simulink library "SMXL"  (Simulink 2.3)
libraries: smxl x55, SMXL x9, simulink3 x4
(part 1 of 2)
settings Model: LastModifiedBy=campa

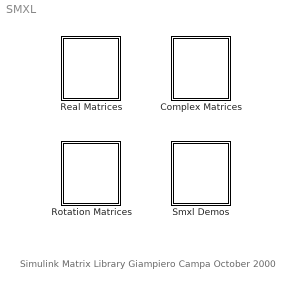
== system SMXL ==
  note: Simulink Matrix Library
      | Giampiero Campa
      | October 2000
  Complex Matrices : Subsystem
      mask Display: disp('Complex\nMatrices')
  Real Matrices : Subsystem
      mask Display: disp('Real\nMatrices')
  Rotation Matrices : Subsystem
      mask Display: disp('R3\nRotation\nMatrices')
  Smxl Demos : Subsystem
      settings: OpenFcn=smxlexamplespath=which('smxl');path(path,[ smxlexamplespath(1:length(smxlexamplespath)-8) 'examples' ]);clear smxlexamplespath;smxldemo
      mask Display: disp('Smxl\nDemos')

== system SMXL/Complex Matrices ==
  note: COMPLEX (AND REAL) MATRICES
  note: Multiplication, Transposition, Pseudoinversion, Rank, Pseudo Singular Values Decomposition
  note: Horizontal Composition, Horizontal Split, Vertical Composition, Vertical Split
  vchcomp : Subsystem  mask(Simulink Matrix Library Block){dims=[3 2 2]}
      mask prompts: dims "[p n m]"
      mask help:
      | Complex Varying Matrices Horizontal Composition
      |   Input 1   : elements of matrix X (p by n)
      |   Input 2   : elements of matrix Y (p by m)
      |   Output   : elements of matrix [X Y] (p by m+n)
      mask Help:
      | <p>
      | Elements of input and output matrices are taken columnwise.
      | </p>
      | <p>
      | To use this block you should have the smxl library in your path.
      | </p>
      mask Display: disp('Z=[X,Y]')
  vchsplit : Subsystem  mask(Simulink Matrix Library Block){dims=[3 2 2]}
      mask prompts: dims "[p n m]"
      mask help:
      | Complex Varying Matrix Horizontal Split
      |   Input       : elements of matrix [X Y] (p by n+m)
      |   Output 1 : elements of matrix X (p by n)
      |   Output 2 : elements of matrix Y (p by m)
      mask Help:
      | <p>
      | Elements of input and output matrices are taken columnwise.
      | </p>
      | <p>
      | To use this block you should have the smxl library in your path.
      | </p>
      mask Display: disp('[X,Y]=Z')
  vcmult : Subsystem  mask(Simulink Matrix Library Block){d=[2 3 2]}
      mask prompts: d "[n p m]"
      mask help:
      | Complex Varying Matrices Multiplication
      |   Input 1   : elements of matrix X (n by p)
      |   Input 2   : elements of matrix Y (p by m)
      |   Output   : elements of matrix X*Y (n by m)
      mask Help:
      | <p>
      | Elements of input and output matrices are taken columnwise.
      | </p>
      | <p>
      | To use this block you should have the smxl library in your path.
      | </p>
      mask Display: disp('Z=X*Y')
  vcpinv : Subsystem  mask(Simulink Matrix Library Block){d=[3 2], tol=1}
      mask prompts: d "[n m]"
      mask help:
      | Complex Varying Matrix Pseudoinversion
      |   Input      : elements of matrix X (n by m)
      |   Output   : elements of matrix Pinv(X) (m by n)
      |   Tol         : tolerance is set to max(m,n)*max(svd(X))*eps*tol
      mask Help:
      | <p>
      | Elements of input and output matrices are taken columnwise.
      | </p>
      | <p>
      | To use this block you should have the smxl library in your path.
      | </p>
      mask Display: disp('Y=pinv(X)')
  vcpsvd : Subsystem  mask(Simulink Matrix Library Block){d=[2 3]}
      mask prompts: d "[n m]"
      mask help:
      | Complex Varying Matrix SVD
      |   Input       : elements of matrix X=USV', (n by m)
      |   Output 1 : elements of matrix U, (n by min(n,m))
      |   Output 2 : elements of matrix S, (square min(n,m))
      |   Output 3 : elements of matrix V, (m by min(n,m))
      |
      |   NOTE     : This is actually a pseudo-svd, since each singular value is
      |                     repeated twice along S diagonal. To have a pure svd just
      |                     pick up every singular value once with the respective
      |                     left and right singular vectors multiplied by sqrt(2).
      mask Help:
      | <p>
      | Elements of input and output matrices are taken columnwise.
      | </p>
      | <p>
      | NOTE     : This is actually a pseudo-svd, since each singular value is
      |                   repeated twice along S diagonal. To have a pure svd just
      |                   pick up every singular value once with the respective
      |                   left and right singular vectors multiplied by sqrt(2).
      | 
      | </p>
      | <p>
      | To use this block you should have the smxl library in your path.
      | </p>
      mask Display: disp('[U,S,V]=svd(X)')
  vcrank : Subsystem  mask(Simulink Matrix Library Block){d=[4 3], tol=1}
      mask prompts: d "[n m]"
      mask help:
      | Complex Varying Matrix Rank
      |   Input      : elements of matrix X (n by m)
      |   Output   : rank of matrix X
      |   Tol         : tolerance is set to max(m,n)*max(svd(X))*eps*tol
      mask Help:
      | <p>
      | Elements of input and output matrices are taken columnwise.
      | </p>
      | <p>
      | To use this block you should have the smxl library in your path.
      | </p>
      mask Display: disp('rank(X)')
  vctrsp : Subsystem  mask(Simulink Matrix Library Block){d=[3 2], h=on}
      mask prompts: d "[n m]"; h "Hermitian"
      mask help:
      | Complex Varying Matrix Transposition
      |   Input      : elements of matrix X (n by m)
      |   Output   : elements of matrix X' (m by n)
      mask Help:
      | <p>
      | Elements of input and output matrices are taken columnwise.
      | </p>
      | <p>
      | To use this block you should have the smxl library in your path.
      | </p>
      mask Display: disp('Y=X''')
  vcvcomp : Subsystem  mask(Simulink Matrix Library Block){dims=[3 3 2]}
      mask prompts: dims "[n m p]"
      mask help:
      | Complex Varying Matrices Vertical Composition
      |   Input 1 : elements of matrix X (n by p)
      |   Input 2 : elements of matrix Y (m by p)
      |   Output : elements of matrix [X;Y] (m+n by p)
      mask Help:
      | <p>
      | Elements of input and output matrices are taken columnwise.
      | </p>
      | <p>
      | To use this block you should have the smxl library in your path.
      | </p>
      mask Display: disp('Z=[X;Y]')
  vcvsplit : Subsystem  mask(Simulink Matrix Library Block){dims=[3 3 2]}
      mask prompts: dims "[n m p]"
      mask help:
      | Complex Varying Matrix Vertical Split
      |   Input       : elements of matrix [X;Y] (n+m by p)
      |   Output 1 : elements of matrix X (n by p)
      |   Output 2 : elements of matrix Y (m by p)
      mask Help:
      | <p>
      | Elements of input and output matrices are taken columnwise.
      | </p>
      | <p>
      | To use this block you should have the smxl library in your path.
      | </p>
      mask Display: disp('[X;Y]=Z')

== system SMXL/Real Matrices ==
  note: Multiplication, Transposition, Pseudoinversion, Rank, Singular Values Decomposition
  note: REAL MATRICES ONLY
  note: Horizontal Composition, Horizontal Split, Vertical Composition, Vertical Split
  vrhcomp : Subsystem  mask(Simulink Matrix Library Block){dims=[3 2 2]}
      mask prompts: dims "[p n m]"
      mask help:
      | Real Varying Matrices Horizontal Composition
      |   Input 1   : elements of matrix X (p by n)
      |   Input 2   : elements of matrix Y (p by m)
      |   Output   : elements of matrix [X Y] (p by m+n)
      mask Help:
      | <p>
      | Elements of input and output matrices are taken columnwise.
      | </p>
      | <p>
      | To use this block you should have the smxl library in your path.
      | </p>
      mask Display: disp('Z=[X,Y]')
  vrhsplit : Subsystem  mask(Simulink Matrix Library Block){dims=[3 2 2]}
      mask prompts: dims "[p n m]"
      mask help:
      | Real Varying Matrix Horizontal Split
      |   Input       : elements of matrix [X Y] (p by n+m)
      |   Output 1 : elements of matrix X (p by n)
      |   Output 2 : elements of matrix Y (p by m)
      mask Help:
      | <p>
      | Elements of input and output matrices are taken columnwise.
      | </p>
      | <p>
      | To use this block you should have the smxl library in your path.
      | </p>
      mask Display: disp('[X,Y]=Z')
  vrmult : S-Function  FunctionName=vrmult  Parameters=dims  PortCounts=[]  SFunctionModules=''  mask(Simulink Matrix Library Block){dims=[2 4 3]}
      mask prompts: dims "[n p m]"
      mask help:
      | Real Varying Matrices Multiplication
      |   Input 1   : elements of matrix X (n by p)
      |   Input 2   : elements of matrix Y (p by m)
      |   Output   : elements of matrix X*Y (n by m)
      mask Help:
      | <p>
      | Elements of input and output matrices are taken columnwise.
      | </p>
      | <p>
      | To use this block you should have the smxl library in your path.
      | </p>
      mask Display: disp('Z=X*Y')
  vrpinv : S-Function  FunctionName=vrpinv  Parameters=dims,tol  PortCounts=[]  SFunctionModules=''  mask(Simulink Matrix Library Block){dims=[3 2], tol=1}
      mask prompts: dims "[n m]"
      mask help:
      | Real Varying Matrix Pseudoinversion
      |   Input      : elements of matrix X (n by m)
      |   Output   : elements of matrix Pinv(X) (m by n)
      |   Tol         : tolerance is set to max(m,n)*max(svd(X))*eps*tol
      mask Help:
      | <p>
      | Elements of input and output matrices are taken columnwise.
      | </p>
      | <p>
      | To use this block you should have the smxl library in your path.
      | </p>
      mask Display: disp('Y=pinv(X)')
  vrrank : Subsystem  mask(Simulink Matrix Library Block){dims=[4 3], tol=1}
      mask prompts: dims "[n m]"
      mask help:
      | Real Varying Matrix Rank
      |   Input      : elements of matrix X (n by m)
      |   Output   : rank of matrix X
      |   Tol         : tolerance is set to max(m,n)*max(svd(X))*eps*tol
      mask Help:
      | <p>
      | Elements of input and output matrices are taken columnwise.
      | </p>
      | <p>
      | To use this block you should have the smxl library in your path.
      | </p>
      mask Display: disp('rank(X)')
  vrsvd : S-Function  FunctionName=vrsvd  Parameters=dims  PortCounts=[]  SFunctionModules=''  mask(Simulink Matrix Library Block){dims=[2 3]}
      mask prompts: dims "[n m]"
      mask help:
      | Real Varying Matrix SVD
      |   Input       : elements of matrix X=USV', (n by m)
      |   Output 1 : elements of matrix U, (n by min(n,m))
      |   Output 2 : elements of matrix S, (square min(n,m))
      |   Output 3 : elements of matrix V, (m by min(n,m))
      mask Help:
      | <p>
      | Elements of input and output matrices are taken columnwise.
      | </p>
      | <p>
      | To use this block you should have the smxl library in your path.
      | </p>
      mask Display: disp('[U,S,V]=svd(X)')
  vrtrsp : Subsystem  mask(Simulink Matrix Library Block){dims=[3 2]}
      mask prompts: dims "[n m]"
      mask help:
      | Real Varying Matrix Transposition
      |   Input      : elements of matrix X (n by m)
      |   Output   : elements of matrix X' (m by n)
      mask Help:
      | <p>
      | Elements of input and output matrices are taken columnwise.
      | </p>
      | <p>
      | To use this block you should have the smxl library in your path.
      | </p>
      mask Display: disp('Y=X''')
  vrvcomp : Subsystem  mask(Simulink Matrix Library Block){dims=[3 3 2]}
      mask prompts: dims "[n m p]"
      mask help:
      | Real Varying Matrices Vertical Composition
      |   Input 1 : elements of matrix X (n by p)
      |   Input 2 : elements of matrix Y (m by p)
      |   Output : elements of matrix [X;Y] (m+n by p)
      mask Help:
      | <p>
      | Elements of input and output matrices are taken columnwise.
      | </p>
      | <p>
      | To use this block you should have the smxl library in your path.
      | </p>
      mask Display: disp('Z=[X;Y]')
  vrvsplit : Subsystem  mask(Simulink Matrix Library Block){dims=[3 3 2]}
      mask prompts: dims "[n m p]"
      mask help:
      | Real Varying Matrix Vertical Split
      |   Input       : elements of matrix [X;Y] (n+m by p)
      |   Output 1 : elements of matrix X (n by p)
      |   Output 2 : elements of matrix Y (m by p)
      mask Help:
      | <p>
      | Elements of input and output matrices are taken columnwise.
      | </p>
      | <p>
      | To use this block you should have the smxl library in your path.
      | </p>
      mask Display: disp('[X;Y]=Z')

== system SMXL/Rotation Matrices ==
  note: Rotation Matrices Library
      | G. Campa & F. Giulietti
      | February 1999
  Euler : Subsystem
      mask Display: disp('Euler')
  Quaternions : Subsystem
      mask Display: disp('Quat')

== system SMXL/Smxl Demos ==

== system SMXL/Complex Matrices/vchcomp ==
  In1 : Inport  Port=1  PortWidth=-1  SampleTime=-1  DataType=auto
      settings: SignalType=auto
  In2 : Inport  Port=2  PortWidth=-1  SampleTime=-1  DataType=auto
      settings: SignalType=auto
  Mux : Mux  Inputs=[dims(1)*dims(2) dims(1)*dims(3)]
  Out1 : Outport  Port=1
  wires:
  In1/1 -> Mux/1
  Mux/1 -> Out1/1
  In2/1 -> Mux/2

== system SMXL/Complex Matrices/vchsplit ==
  In1 : Inport  Port=1  PortWidth=-1  SampleTime=-1  DataType=auto
      settings: SignalType=auto
  Demux : Demux  Outputs=[dims(1)*dims(2) dims(1)*dims(3)]
  Out1 : Outport  Port=1
  Out2 : Outport  Port=2
  wires:
  In1/1 -> Demux/1
  Demux/2 -> Out2/1
  Demux/1 -> Out1/1

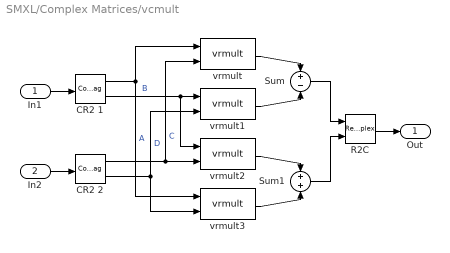
== system SMXL/Complex Matrices/vcmult ==
  In1 : Inport  Port=1  PortWidth=-1  SampleTime=-1  DataType=auto
      settings: SignalType=auto
  In2 : Inport  Port=2  PortWidth=-1  SampleTime=-1  DataType=auto
      settings: SignalType=auto
  CR2 1 : ComplexToRealImag  Output=RealAndImag
  CR2 2 : ComplexToRealImag  Output=RealAndImag
  R2C : RealImagToComplex  Input=RealAndImag  ConstantPart=0
  Sum : Sum  Inputs=+|-  SaturateOnIntegerOverflow=on
  Sum1 : Sum  Inputs=+|+  SaturateOnIntegerOverflow=on
  vrmult{,1..3} (4 alike) : smxl/Real Matrices/vrmult  dims=d
  Out : Outport  Port=1
  wires:
  CR2 1/1 -> vrmult/1, vrmult3/1  "A"
  CR2 1/2 -> vrmult1/1, vrmult2/1  "B"
  CR2 2/2 -> vrmult3/2, vrmult1/2  "D"
  CR2 2/1 -> vrmult2/2, vrmult/2  "C"
  Sum/1 -> R2C/1
  Sum1/1 -> R2C/2
  In1/1 -> CR2 1/1
  R2C/1 -> Out/1
  In2/1 -> CR2 2/1
  vrmult3/1 -> Sum1/2
  vrmult2/1 -> Sum1/1
  vrmult1/1 -> Sum/2
  vrmult/1 -> Sum/1

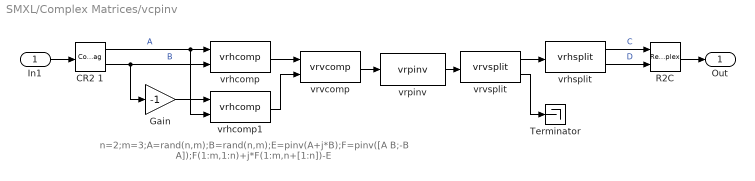
== system SMXL/Complex Matrices/vcpinv ==
  note: n=2;m=3;A=rand(n,m);B=rand(n,m);E=pinv(A+j*B);F=pinv([A B;-B A]);F(1:m,1:n)+j*F(1:m,n+[1:n])-E
  In1 : Inport  Port=1  PortWidth=-1  SampleTime=-1  DataType=auto
      settings: SignalType=auto
  CR2 1 : ComplexToRealImag  Output=RealAndImag
  Gain : Gain  Gain=-1  SaturateOnIntegerOverflow=on
  R2C : RealImagToComplex  Input=RealAndImag  ConstantPart=0
  Terminator : Terminator
  vrhcomp : smxl/Real Matrices/vrhcomp  dims=[d(1) d(2) d(2)]
  vrhcomp1 : smxl/Real Matrices/vrhcomp  dims=[d(1) d(2) d(2)]
  vrhsplit : smxl/Real Matrices/vrhsplit  dims=[d(2) d(1) d(1)]
  vrpinv : smxl/Real Matrices/vrpinv  dims=2*d  tol=tol
  vrvcomp : smxl/Real Matrices/vrvcomp  dims=[d(1) d(1) 2*d(2)]
  vrvsplit : smxl/Real Matrices/vrvsplit  dims=[d(2) d(2) 2*d(1)]
  Out : Outport  Port=1
  wires:
  In1/1 -> CR2 1/1
  CR2 1/1 -> vrhcomp/1, vrhcomp1/2  "A"
  CR2 1/2 -> vrhcomp/2, Gain/1  "B"
  vrhcomp/1 -> vrvcomp/1
  vrhcomp1/1 -> vrvcomp/2
  vrvcomp/1 -> vrpinv/1
  vrpinv/1 -> vrvsplit/1
  vrvsplit/1 -> vrhsplit/1
  vrhsplit/1 -> R2C/1  "C"
  vrhsplit/2 -> R2C/2  "D"
  vrvsplit/2 -> Terminator/1
  Gain/1 -> vrhcomp1/1
  R2C/1 -> Out/1

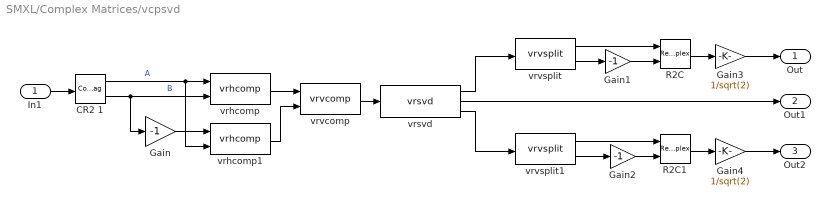
== system SMXL/Complex Matrices/vcpsvd ==
  In1 : Inport  Port=1  PortWidth=-1  SampleTime=-1  DataType=auto
      settings: SignalType=auto
  CR2 1 : ComplexToRealImag  Output=RealAndImag
  Gain : Gain  Gain=-1  SaturateOnIntegerOverflow=on
  Gain1 : Gain  Gain=-1  SaturateOnIntegerOverflow=on
  Gain2 : Gain  Gain=-1  SaturateOnIntegerOverflow=on
  Gain3 : Gain  Gain=1/sqrt(2)  SaturateOnIntegerOverflow=on
  Gain4 : Gain  Gain=1/sqrt(2)  SaturateOnIntegerOverflow=on
  R2C : RealImagToComplex  Input=RealAndImag  ConstantPart=0
  R2C1 : RealImagToComplex  Input=RealAndImag  ConstantPart=0
  vrhcomp : smxl/Real Matrices/vrhcomp  dims=[d(1) d(2) d(2)]
  vrhcomp1 : smxl/Real Matrices/vrhcomp  dims=[d(1) d(2) d(2)]
  vrsvd : smxl/Real Matrices/vrsvd  dims=2*d
  vrvcomp : smxl/Real Matrices/vrvcomp  dims=[d(1) d(1) 2*d(2)]
  vrvsplit : smxl/Real Matrices/vrvsplit  dims=[d(1) d(1) 2*min(d(1),d(2))]
  vrvsplit1 : smxl/Real Matrices/vrvsplit  dims=[d(2) d(2) 2*min(d(1),d(2))]
  Out : Outport  Port=1
  Out1 : Outport  Port=2
  Out2 : Outport  Port=3
  wires:
  In1/1 -> CR2 1/1
  CR2 1/1 -> vrhcomp/1, vrhcomp1/2  "A"
  CR2 1/2 -> vrhcomp/2, Gain/1  "B"
  vrvcomp/1 -> vrsvd/1
  Gain/1 -> vrhcomp1/1
  vrsvd/2 -> Out1/1
  vrsvd/1 -> vrvsplit/1
  vrvsplit/2 -> Gain1/1
  Gain1/1 -> R2C/2
  vrvsplit/1 -> R2C/1
  vrsvd/3 -> vrvsplit1/1
  vrvsplit1/2 -> Gain2/1
  Gain2/1 -> R2C1/2
  vrvsplit1/1 -> R2C1/1
  R2C/1 -> Gain3/1
  Gain3/1 -> Out/1
  R2C1/1 -> Gain4/1
  Gain4/1 -> Out2/1
  vrhcomp/1 -> vrvcomp/1
  vrhcomp1/1 -> vrvcomp/2

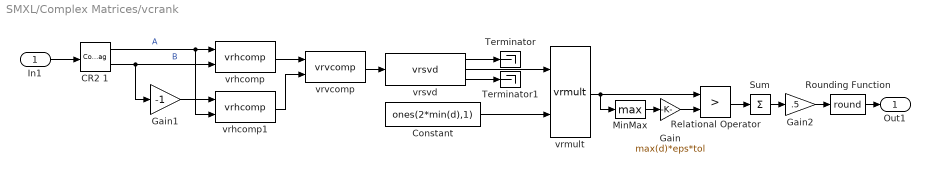
== system SMXL/Complex Matrices/vcrank ==
  In1 : Inport  Port=1  PortWidth=-1  SampleTime=-1  DataType=auto
      settings: SignalType=auto
  CR2 1 : ComplexToRealImag  Output=RealAndImag
  Constant : Constant  Value=ones(2*min(d),1)
  Gain : Gain  Gain=max(d)*eps*tol  SaturateOnIntegerOverflow=on
  Gain1 : Gain  Gain=-1  SaturateOnIntegerOverflow=on
  Gain2 : Gain  Gain=.5  SaturateOnIntegerOverflow=on
  MinMax : MinMax  Function=max  Inputs=1
  Relational Operator : RelationalOperator  Operator=>
  Rounding Function : Rounding  Operator=round
  Sum : Sum  Inputs=1  SaturateOnIntegerOverflow=on
  Terminator : Terminator
  Terminator1 : Terminator
  vrhcomp : smxl/Real Matrices/vrhcomp  dims=[d(1) d(2) d(2)]
  vrhcomp1 : smxl/Real Matrices/vrhcomp  dims=[d(1) d(2) d(2)]
  vrmult : smxl/Real Matrices/vrmult  dims=[2*min(d) 2*min(d) 1]
  vrsvd : smxl/Real Matrices/vrsvd  dims=2*d
  vrvcomp : smxl/Real Matrices/vrvcomp  dims=[d(1) d(1) 2*d(2)]
  Out1 : Outport  Port=1
  wires:
  CR2 1/2 -> vrhcomp/2, Gain1/1  "B"
  CR2 1/1 -> vrhcomp/1, vrhcomp1/2  "A"
  In1/1 -> CR2 1/1
  Gain1/1 -> vrhcomp1/1
  vrvcomp/1 -> vrsvd/1
  Gain/1 -> Relational Operator/2
  MinMax/1 -> Gain/1
  vrmult/1 -> MinMax/1, Relational Operator/1
  vrsvd/2 -> vrmult/1
  Constant/1 -> vrmult/2
  vrsvd/3 -> Terminator1/1
  vrsvd/1 -> Terminator/1
  Relational Operator/1 -> Sum/1
  Rounding Function/1 -> Out1/1
  Gain2/1 -> Rounding Function/1
  Sum/1 -> Gain2/1
  vrhcomp1/1 -> vrvcomp/2
  vrhcomp/1 -> vrvcomp/1

== system SMXL/Complex Matrices/vctrsp ==
  In1 : Inport  Port=1  PortWidth=-1  SampleTime=-1  DataType=auto
      settings: SignalType=auto
  CR2 1 : ComplexToRealImag  Output=RealAndImag
  Gain : Gain  Gain=1-2*h  SaturateOnIntegerOverflow=on
  R2C : RealImagToComplex  Input=RealAndImag  ConstantPart=0
  vrtrsp : smxl/Real Matrices/vrtrsp  dims=d
  vrtrsp1 : smxl/Real Matrices/vrtrsp  dims=d
  Out : Outport  Port=1
  wires:
  In1/1 -> CR2 1/1
  CR2 1/2 -> vrtrsp1/1  "B"
  CR2 1/1 -> vrtrsp/1  "A"
  R2C/1 -> Out/1
  vrtrsp/1 -> R2C/1
  vrtrsp1/1 -> Gain/1
  Gain/1 -> R2C/2

== system SMXL/Complex Matrices/vcvcomp ==
  In1 : Inport  Port=1  PortWidth=-1  SampleTime=-1  DataType=auto
      settings: SignalType=auto
  In2 : Inport  Port=2  PortWidth=-1  SampleTime=-1  DataType=auto
      settings: SignalType=auto
  Mux : Mux  Inputs=[dims(3)*dims(1) dims(3)*dims(2)]
  vctrsp : smxl/Complex Matrices/vctrsp  d=[dims(1) dims(3)]  h=on
  vctrsp1 : smxl/Complex Matrices/vctrsp  d=[dims(2) dims(3)]  h=on
  vctrsp2 : smxl/Complex Matrices/vctrsp  d=[dims(3) dims(2)+dims(1)]  h=on
  Out1 : Outport  Port=1
  wires:
  In1/1 -> vctrsp/1
  In2/1 -> vctrsp1/1
  vctrsp2/1 -> Out1/1
  Mux/1 -> vctrsp2/1
  vctrsp1/1 -> Mux/2
  vctrsp/1 -> Mux/1

== system SMXL/Complex Matrices/vcvsplit ==
  In1 : Inport  Port=1  PortWidth=-1  SampleTime=-1  DataType=auto
      settings: SignalType=auto
  Demux : Demux  Outputs=[dims(3)*dims(1) dims(3)*dims(2)]
  vctrsp : smxl/Complex Matrices/vctrsp  d=[dims(3) dims(1)]  h=on
  vctrsp1 : smxl/Complex Matrices/vctrsp  d=[dims(3) dims(2)]  h=on
  vctrsp2 : smxl/Complex Matrices/vctrsp  d=[dims(2)+dims(1) dims(3)]  h=on
  Out1 : Outport  Port=1
  Out2 : Outport  Port=2
  wires:
  In1/1 -> vctrsp2/1
  vctrsp2/1 -> Demux/1
  Demux/1 -> vctrsp/1
  vctrsp/1 -> Out1/1
  Demux/2 -> vctrsp1/1
  vctrsp1/1 -> Out2/1

== system SMXL/Real Matrices/vrhcomp ==
  In1 : Inport  Port=1  PortWidth=-1  SampleTime=-1  DataType=auto
      settings: SignalType=auto
  In2 : Inport  Port=2  PortWidth=-1  SampleTime=-1  DataType=auto
      settings: SignalType=auto
  Mux : Mux  Inputs=[dims(1)*dims(2) dims(1)*dims(3)]
  Out1 : Outport  Port=1
  wires:
  In2/1 -> Mux/2
  Mux/1 -> Out1/1
  In1/1 -> Mux/1

== system SMXL/Real Matrices/vrhsplit ==
  In1 : Inport  Port=1  PortWidth=-1  SampleTime=-1  DataType=auto
      settings: SignalType=auto
  Demux : Demux  Outputs=[dims(1)*dims(2) dims(1)*dims(3)]
  Out1 : Outport  Port=1
  Out2 : Outport  Port=2
  wires:
  Demux/1 -> Out1/1
  Demux/2 -> Out2/1
  In1/1 -> Demux/1

== system SMXL/Real Matrices/vrrank ==
  In1 : Inport  Port=1  PortWidth=-1  SampleTime=-1  DataType=auto
      settings: SignalType=auto
  Constant : Constant  Value=ones(min(dims),1)
  Gain : Gain  Gain=max(dims)*eps*tol  SaturateOnIntegerOverflow=on
  MinMax : MinMax  Function=max  Inputs=1
  Relational Operator : RelationalOperator  Operator=>
  Sum : Sum  Inputs=1  SaturateOnIntegerOverflow=on
  Terminator : Terminator
  Terminator1 : Terminator
  vrmult : SMXL/Real Matrices/vrmult  dims=[min(dims) min(dims) 1]
  vrsvd : SMXL/Real Matrices/vrsvd  dims=dims
  Out1 : Outport  Port=1
  wires:
  vrsvd/1 -> Terminator/1
  vrsvd/3 -> Terminator1/1
  Constant/1 -> vrmult/2
  In1/1 -> vrsvd/1
  vrsvd/2 -> vrmult/1
  vrmult/1 -> Relational Operator/1, MinMax/1
  Relational Operator/1 -> Sum/1
  Sum/1 -> Out1/1
  MinMax/1 -> Gain/1
  Gain/1 -> Relational Operator/2

== system SMXL/Real Matrices/vrtrsp ==
  In : Inport  Port=1  PortWidth=-1  SampleTime=-1  DataType=auto
      settings: SignalType=auto
  Selector : Selector  Elements=reshape(reshape(1:dims(1)*dims(2),dims(1),dims(2))',dims(1)*dims(2),1)  InputPortWidth=dims(1)*dims(2)
  Out : Outport  Port=1
  wires:
  Selector/1 -> Out/1
  In/1 -> Selector/1

== system SMXL/Real Matrices/vrvcomp ==
  In1 : Inport  Port=1  PortWidth=-1  SampleTime=-1  DataType=auto
      settings: SignalType=auto
  In2 : Inport  Port=2  PortWidth=-1  SampleTime=-1  DataType=auto
      settings: SignalType=auto
  Mux : Mux  Inputs=[dims(3)*dims(1) dims(3)*dims(2)]
  vrtrsp : smxl/Real Matrices/vrtrsp  dims=[dims(1) dims(3)]
  vrtrsp1 : smxl/Real Matrices/vrtrsp  dims=[dims(2) dims(3)]
  vrtrsp2 : smxl/Real Matrices/vrtrsp  dims=[dims(3) dims(2)+dims(1)]
  Out1 : Outport  Port=1
  wires:
  vrtrsp/1 -> Mux/1
  vrtrsp1/1 -> Mux/2
  Mux/1 -> vrtrsp2/1
  vrtrsp2/1 -> Out1/1
  In2/1 -> vrtrsp1/1
  In1/1 -> vrtrsp/1

== system SMXL/Real Matrices/vrvsplit ==
  In1 : Inport  Port=1  PortWidth=-1  SampleTime=-1  DataType=auto
      settings: SignalType=auto
  Demux : Demux  Outputs=[dims(3)*dims(1) dims(3)*dims(2)]
  vrtrsp : smxl/Real Matrices/vrtrsp  dims=[dims(3) dims(1)]
  vrtrsp1 : smxl/Real Matrices/vrtrsp  dims=[dims(3) dims(2)]
  vrtrsp2 : smxl/Real Matrices/vrtrsp  dims=[dims(2)+dims(1) dims(3)]
  Out1 : Outport  Port=1
  Out2 : Outport  Port=2
  wires:
  vrtrsp1/1 -> Out2/1
  Demux/2 -> vrtrsp1/1
  vrtrsp/1 -> Out1/1
  Demux/1 -> vrtrsp/1
  vrtrsp2/1 -> Demux/1
  In1/1 -> vrtrsp2/1

== system SMXL/Rotation Matrices/Euler ==
  Body2Earth : Subsystem
      mask Type: Simulink Matrix Library Block
      mask Description:
      | Rotation matrix from Body to Earth :
      |   Input 1 : Roll, Pitch and Yaw angles (phi,theta,psi)
      |   Input 2 : V (3 by 1) vector in Body coordinates
      |   Output : V (3 by 1) vector in Earth coordinates
      mask Help:
      | <p>
      | Roll, Pitch and Yaw angles express the orientation
      | of the Body frame with respect to the Earth frame.
      | </p>
      | <p>
      | To use this block you should have the smxl library in your path.
      | </p>
  Body2Wind : Subsystem
      mask Type: Simulink Matrix Library Block
      mask Description:
      | Rotation matrix from Body to Wind :
      |   Input 1 : Attack and Sideslip angles (alpha and beta)
      |   Input 2 : V (3 by 1) vector in Body coordinates
      |   Output : V (3 by 1) vector in Wind coordinates
      mask Help:
      | <p>
      | Attack and Sideslip angles express the orientation
      | of the Wind frame with respect to the Body frame.
      | </p>
      | <p>
      | To use this block you should have the smxl library in your path.
      | </p>
  Earth2Body : Subsystem
      mask Type: Simulink Matrix Library Block
      mask Description:
      | Rotation matrix from Earth to Body :
      |   Input 1 : Roll, Pitch and Yaw angles (phi,theta,psi)
      |   Input 2 : V (3 by 1) vector in Earth coordinates
      |   Output : V (3 by 1) vector in Body coordinates
      mask Help:
      | <p>
      | Roll, Pitch and Yaw angles express the orientation
      | of the Body frame with respect to the Earth frame.
      | </p>
      | <p>
      | To use this block you should have the smxl library in your path.
      | </p>
  Earth2Kine : Subsystem
      mask Type: Simulink Matrix Library Block
      mask Description:
      | Rotation matrix from Earth to Kinematic  :
      |   Input 1 : Heading, Flight Path and Bank angles (Chi, Gamma, Mu)
      |   Input 2 : V (3 by 1) vector in Earth coordinates
      |   Output : V (3 by 1) vector in Kinematic coordinates
      mask Help:
      | <p>
      |  Heading, Flight Path and Bank angles express the orientation
      | of the Kinematic frame with respect to the Earth frame.
      | </p>
      | <p>
      | To use this block you should have the smxl library in your path.
      | </p>
  Kine2Earth : Subsystem
      mask Type: Simulink Matrix Library Block
      mask Description:
      | Rotation matrix from Kinematic to Earth :
      |   Input 1 : Heading, Flight Path and Bank angles (Chi, Gamma, Mu)
      |   Input 2 : V (3 by 1) vector in Kinematic coordinates
      |   Output : V (3 by 1) vector in Earth coordinates
      mask Help:
      | <p>
      |  Heading, Flight Path and Bank angles express the orientation
      | of the Kinematic frame with respect to the Earth frame.
      | </p>
      | <p>
      | To use this block you should have the smxl library in your path.
      | </p>
  Wind2Body : Subsystem
      mask Type: Simulink Matrix Library Block
      mask Description:
      | Rotation matrix from Wind to Body :
      |   Input 1 : Attack and Sideslip angles (alpha and beta)
      |   Input 2 : V (3 by 1) vector in Wind coordinates
      |   Output : V (3 by 1) vector in Body coordinates
      mask Help:
      | <p>
      | Attack and Sideslip angles express the orientation
      | of the Wind frame with respect to the Body frame.
      | </p>
      | <p>
      | To use this block you should have the smxl library in your path.
      | </p>
  ftpdot2pqr : Subsystem
      mask Type: Simulink Matrix Library Block
      mask Description:
      | Roll, Pitch and Yaw derivatives to Omega :
      |   Input 1 : Roll, Pitch and Yaw angles (phi,theta,psi)
      |   Input 2 : Roll, Pitch and Yaw derivatives
      |   Output : Omega (p,q,r)
      mask Help:
      | <p>
      | Roll, Pitch and Yaw angles express the orientation
      | of the Body frame with respect to the Earth frame.
      | </p>
      | <p>
      | To use this block you should have the smxl library in your path.
      | </p>
  pqr2ftpdot : Subsystem
      mask Type: Simulink Matrix Library Block
      mask Description:
      | Omega to Roll, Pitch and Yaw derivatives :
      |   Input 1 : Roll, Pitch and Yaw angles (phi,theta,psi)
      |   Input 2 : Omega (p,q,r)
      |   Output : Roll, Pitch and Yaw derivatives
      mask Help:
      | <p>
      | Roll, Pitch and Yaw angles express the orientation
      | of the Body frame with respect to the Earth frame.
      | </p>
      | <p>
      | To use this block you should have the smxl library in your path.
      | </p>

== system SMXL/Rotation Matrices/Quaternions ==
  Body2Earth : Subsystem
      mask Type: Simulink Matrix Library Block
      mask Description:
      | Rotation matrix from Body to Earth :
      |   Input 1 : Unit Quaternion [q1,q2,q3,q0]
      |   Input 2 : V (3 by 1) vector in Body coordinates
      |   Output : V (3 by 1) vector in Earth coordinates
      mask Help:
      | <p>
      | The Unit Quaternion [q1,q2,q3,q0] express the orientation
      | of the Body frame with respect to the Earth frame.
      | </p>
      | <p>
      | To use this block you should have the smxl library in your path.
      | </p>
  Earth2Body : Subsystem
      mask Type: Simulink Matrix Library Block
      mask Description:
      | Rotation matrix from Earth to Body :
      |   Input 1 : Unit Quaternion [q1,q2,q3,q0]
      |   Input 2 : V (3 by 1) vector in Earth coordinates
      |   Output : V (3 by 1) vector in Body coordinates
      mask Help:
      | <p>
      | The Unit Quaternion [q1,q2,q3,q0] express the orientation
      | of the Body frame with respect to the Earth frame.
      | </p>
      | <p>
      | To use this block you should have the smxl library in your path.
      | </p>
  endot2pqr : Subsystem
      mask Type: Simulink Matrix Library Block
      mask Description:
      | Unit Quaternion derivatives to Omega :
      |   Input 1 : Unit Quaternion [q1,q2,q3,q0]
      |   Input 2 : Unit Quaternion derivatives
      |   Output : Omega (p,q,r)
      mask Help:
      | <p>
      | The Unit Quaternion [q1,q2,q3,q0] express the orientation
      | of the Body frame with respect to the Earth frame.
      | </p>
      | <p>
      | To use this block you should have the smxl library in your path.
      | </p>
  pqr2endot : Subsystem
      mask Type: Simulink Matrix Library Block
      mask Description:
      | Omega to Unit Quaternion derivatives :
      |   Input 1 : Unit Quaternion [q1,q2,q3,q0]
      |   Input 2 : Omega (p,q,r)
      |   Output : Unit Quaternion derivatives
      mask Help:
      | <p>
      | The Unit Quaternion [q1,q2,q3,q0] express the orientation
      | of the Body frame with respect to the Earth frame.
      | </p>
      | <p>
      | To use this block you should have the smxl library in your path.
      | </p>

== system SMXL/Rotation Matrices/Euler/Body2Earth ==
  ftp : Inport  Port=1  PortWidth=-1  SampleTime=-1  DataType=auto
      settings: SignalType=auto
  Vb : Inport  Port=2  PortWidth=-1  SampleTime=-1  DataType=auto
      settings: SignalType=auto
  Demux : Demux  Outputs=3
  Selector : Selector  Elements=[3 2 1]  InputPortWidth=3
  Tcf : Subsystem
  Tfb : Subsystem
  Toc : Subsystem
  vrmult : smxl/Real Matrices/vrmult  dims=[3 3 3]
  vrmult1 : smxl/Real Matrices/vrmult  dims=[3 3 3]
  vrmult2 : smxl/Real Matrices/vrmult  dims=[3 3 1]
  Ve : Outport  Port=1
  wires:
  ftp/1 -> Selector/1
  Demux/1 -> Toc/1(psi)  "psi"
  Demux/2 -> Tcf/1(theta)  "theta"
  Demux/3 -> Tfb/1(phi)  "phi"
  Selector/1 -> Demux/1
  Toc/1(Toc) -> vrmult/1
  Tcf/1(Tcf) -> vrmult/2
  vrmult/1 -> vrmult1/1
  Tfb/1(Tfb) -> vrmult1/2
  vrmult1/1 -> vrmult2/1
  Vb/1 -> vrmult2/2
  vrmult2/1 -> Ve/1

== system SMXL/Rotation Matrices/Euler/Body2Wind ==
  ab : Inport  Port=1  PortWidth=-1  SampleTime=-1  DataType=auto
      settings: SignalType=auto
  Vb : Inport  Port=2  PortWidth=-1  SampleTime=-1  DataType=auto
      settings: SignalType=auto
  Demux1 : Demux  Outputs=2
  Gain : Gain  Gain=-1  SaturateOnIntegerOverflow=on
  Tcf : Subsystem
  Toc : Subsystem
  vrmult : smxl/Real Matrices/vrmult  dims=[3 3 3]
  vrmult2 : smxl/Real Matrices/vrmult  dims=[3 3 1]
  vrtrsp : smxl/Real Matrices/vrtrsp  dims=[3 3]
  Vw : Outport  Port=1
  wires:
  Demux1/1 -> Gain/1  "alpha"
  Gain/1 -> Tcf/1(alpha)
  Demux1/2 -> Toc/1(beta)  "beta"
  Toc/1(Toc) -> vrmult/2
  Tcf/1(Tcf) -> vrmult/1
  ab/1 -> Demux1/1
  vrmult/1 -> vrtrsp/1
  vrmult2/1 -> Vw/1
  vrtrsp/1 -> vrmult2/1
  Vb/1 -> vrmult2/2

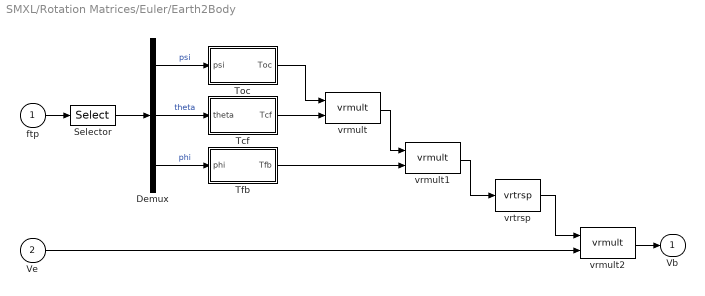
== system SMXL/Rotation Matrices/Euler/Earth2Body ==
  ftp : Inport  Port=1  PortWidth=-1  SampleTime=-1  DataType=auto
      settings: SignalType=auto
  Ve : Inport  Port=2  PortWidth=-1  SampleTime=-1  DataType=auto
      settings: SignalType=auto
  Demux : Demux  Outputs=3
  Selector : Selector  Elements=[3 2 1]  InputPortWidth=3
  Tcf : Subsystem
  Tfb : Subsystem
  Toc : Subsystem
  vrmult : smxl/Real Matrices/vrmult  dims=[3 3 3]
  vrmult1 : smxl/Real Matrices/vrmult  dims=[3 3 3]
  vrmult2 : smxl/Real Matrices/vrmult  dims=[3 3 1]
  vrtrsp : smxl/Real Matrices/vrtrsp  dims=[3 3]
  Vb : Outport  Port=1
  wires:
  vrmult2/1 -> Vb/1
  vrtrsp/1 -> vrmult2/1
  Ve/1 -> vrmult2/2
  vrmult1/1 -> vrtrsp/1
  Tfb/1(Tfb) -> vrmult1/2
  vrmult/1 -> vrmult1/1
  Tcf/1(Tcf) -> vrmult/2
  Toc/1(Toc) -> vrmult/1
  Selector/1 -> Demux/1
  Demux/3 -> Tfb/1(phi)  "phi"
  Demux/2 -> Tcf/1(theta)  "theta"
  Demux/1 -> Toc/1(psi)  "psi"
  ftp/1 -> Selector/1

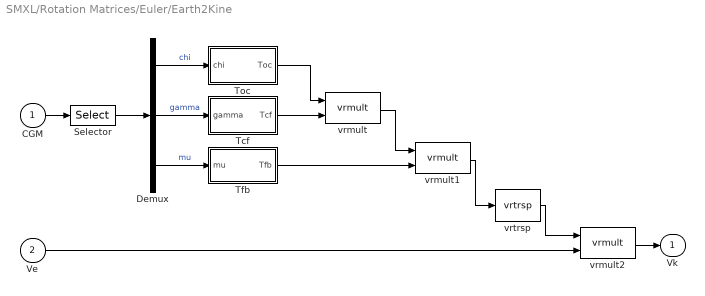
== system SMXL/Rotation Matrices/Euler/Earth2Kine ==
  CGM : Inport  Port=1  PortWidth=-1  SampleTime=-1  DataType=auto
      settings: SignalType=auto
  Ve : Inport  Port=2  PortWidth=-1  SampleTime=-1  DataType=auto
      settings: SignalType=auto
  Demux : Demux  Outputs=3
  Selector : Selector  Elements=[3 2 1]  InputPortWidth=3
  Tcf : Subsystem
  Tfb : Subsystem
  Toc : Subsystem
  vrmult : SMXL/Real Matrices/vrmult  dims=[3 3 3]
  vrmult1 : SMXL/Real Matrices/vrmult  dims=[3 3 3]
  vrmult2 : SMXL/Real Matrices/vrmult  dims=[3 3 1]
  vrtrsp : SMXL/Real Matrices/vrtrsp  dims=[3 3]
  Vk : Outport  Port=1
  wires:
  Demux/1 -> Toc/1(chi)  "chi"
  Demux/2 -> Tcf/1(gamma)  "gamma"
  Demux/3 -> Tfb/1(mu)  "mu"
  Toc/1(Toc) -> vrmult/1
  Tcf/1(Tcf) -> vrmult/2
  vrmult/1 -> vrmult1/1
  Tfb/1(Tfb) -> vrmult1/2
  vrmult1/1 -> vrtrsp/1
  vrmult2/1 -> Vk/1
  vrtrsp/1 -> vrmult2/1
  Ve/1 -> vrmult2/2
  Selector/1 -> Demux/1
  CGM/1 -> Selector/1

== system SMXL/Rotation Matrices/Euler/Kine2Earth ==
  CGM : Inport  Port=1  PortWidth=-1  SampleTime=-1  DataType=auto
      settings: SignalType=auto
  Vk : Inport  Port=2  PortWidth=-1  SampleTime=-1  DataType=auto
      settings: SignalType=auto
  Demux : Demux  Outputs=3
  Selector : Selector  Elements=[3 2 1]  InputPortWidth=3
  Tcf : Subsystem
  Tfb : Subsystem
  Toc : Subsystem
  vrmult : SMXL/Real Matrices/vrmult  dims=[3 3 3]
  vrmult1 : SMXL/Real Matrices/vrmult  dims=[3 3 3]
  vrmult2 : SMXL/Real Matrices/vrmult  dims=[3 3 1]
  Ve : Outport  Port=1
  wires:
  CGM/1 -> Selector/1
  Demux/1 -> Toc/1(chi)  "chi"
  Demux/2 -> Tcf/1(gamma)  "gamma"
  Demux/3 -> Tfb/1(mu)  "mu"
  Selector/1 -> Demux/1
  Toc/1(Toc) -> vrmult/1
  Tcf/1(Tcf) -> vrmult/2
  vrmult/1 -> vrmult1/1
  Tfb/1(Tfb) -> vrmult1/2
  vrmult1/1 -> vrmult2/1
  Vk/1 -> vrmult2/2
  vrmult2/1 -> Ve/1

== system SMXL/Rotation Matrices/Euler/Wind2Body ==
  ab : Inport  Port=1  PortWidth=-1  SampleTime=-1  DataType=auto
      settings: SignalType=auto
  Vw : Inport  Port=2  PortWidth=-1  SampleTime=-1  DataType=auto
      settings: SignalType=auto
  Demux1 : Demux  Outputs=2
  Gain : Gain  Gain=-1  SaturateOnIntegerOverflow=on
  Tcf : Subsystem
  Toc : Subsystem
  vrmult : smxl/Real Matrices/vrmult  dims=[3 3 3]
  vrmult2 : smxl/Real Matrices/vrmult  dims=[3 3 1]
  Vb : Outport  Port=1
  wires:
  Demux1/1 -> Gain/1  "alpha"
  Gain/1 -> Tcf/1(alpha)
  Demux1/2 -> Toc/1(beta)  "beta"
  Toc/1(Toc) -> vrmult/2
  Tcf/1(Tcf) -> vrmult/1
  vrmult2/1 -> Vb/1
  vrmult/1 -> vrmult2/1
  ab/1 -> Demux1/1
  Vw/1 -> vrmult2/2

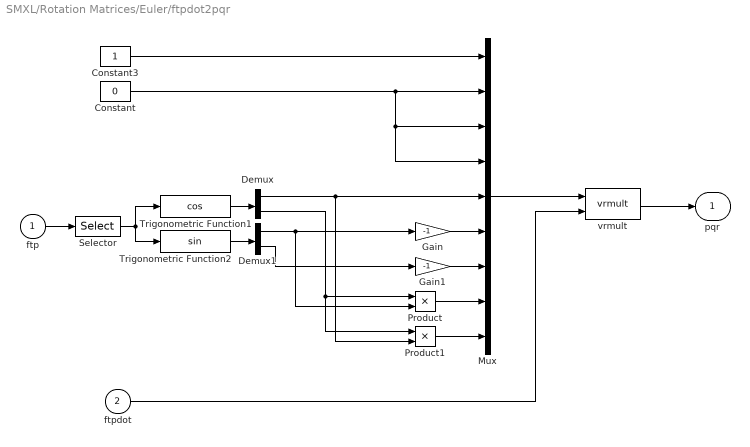
== system SMXL/Rotation Matrices/Euler/ftpdot2pqr ==
  ftp : Inport  Port=1  PortWidth=-1  SampleTime=-1  DataType=auto
      settings: SignalType=auto
  ftpdot : Inport  Port=2  PortWidth=-1  SampleTime=-1  DataType=auto
      settings: SignalType=auto
  Constant : Constant  Value=0
  Constant3 : Constant  Value=1
  Demux : Demux  Outputs=2
  Demux1 : Demux  Outputs=2
  Gain : Gain  Gain=-1  SaturateOnIntegerOverflow=on
  Gain1 : Gain  Gain=-1  SaturateOnIntegerOverflow=on
  Mux : Mux  Inputs=9
  Product : Product  Inputs=2  SaturateOnIntegerOverflow=on
  Product1 : Product  Inputs=2  SaturateOnIntegerOverflow=on
  Selector : Selector  Elements=[1 2]  InputPortWidth=3
  Trigonometric Function1 : Trigonometry  Operator=cos  OutputSignalType=auto
  Trigonometric Function2 : Trigonometry  Operator=sin  OutputSignalType=auto
  vrmult : smxl/Real Matrices/vrmult  dims=[3 3 1]
  pqr : Outport  Port=1
  wires:
  ftp/1 -> Selector/1
  Demux1/1 -> Product/2, Gain/1
  Trigonometric Function2/1 -> Demux1/1
  vrmult/1 -> pqr/1
  Mux/1 -> vrmult/1
  ftpdot/1 -> vrmult/2
  Selector/1 -> Trigonometric Function2/1, Trigonometric Function1/1
  Demux/1 -> Product1/2, Mux/5
  Demux/2 -> Product1/1, Product/1
  Product1/1 -> Mux/9
  Product/1 -> Mux/8
  Demux1/2 -> Gain1/1
  Trigonometric Function1/1 -> Demux/1
  Gain1/1 -> Mux/7
  Gain/1 -> Mux/6
  Constant/1 -> Mux/4, Mux/3, Mux/2
  Constant3/1 -> Mux/1

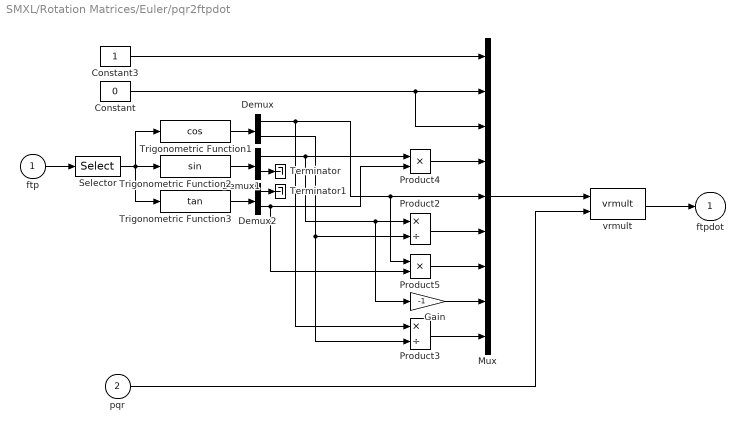
== system SMXL/Rotation Matrices/Euler/pqr2ftpdot ==
  ftp : Inport  Port=1  PortWidth=-1  SampleTime=-1  DataType=auto
      settings: SignalType=auto
  pqr : Inport  Port=2  PortWidth=-1  SampleTime=-1  DataType=auto
      settings: SignalType=auto
  Constant : Constant  Value=0
  Constant3 : Constant  Value=1
  Demux : Demux  Outputs=2
  Demux1 : Demux  Outputs=2
  Demux2 : Demux  Outputs=2
  Gain : Gain  Gain=-1  SaturateOnIntegerOverflow=on
  Mux : Mux  Inputs=9
  Product2 : Product  Inputs=*/  SaturateOnIntegerOverflow=on
  Product3 : Product  Inputs=*/  SaturateOnIntegerOverflow=on
  Product4 : Product  Inputs=2  SaturateOnIntegerOverflow=on
  Product5 : Product  Inputs=2  SaturateOnIntegerOverflow=on
  Selector : Selector  Elements=[1 2]  InputPortWidth=3
  Terminator : Terminator
  Terminator1 : Terminator
  Trigonometric Function1 : Trigonometry  Operator=cos  OutputSignalType=auto
  Trigonometric Function2 : Trigonometry  Operator=sin  OutputSignalType=auto
  Trigonometric Function3 : Trigonometry  Operator=tan  OutputSignalType=auto
  vrmult : smxl/Real Matrices/vrmult  dims=[3 3 1]
  ftpdot : Outport  Port=1
  wires:
  Gain/1 -> Mux/8
  Demux2/1 -> Terminator1/1
  Demux1/2 -> Terminator/1
  Product3/1 -> Mux/9
  Demux/2 -> Product3/2, Product2/2
  Demux/1 -> Product3/1, Product5/1, Mux/5
  Demux2/2 -> Product5/2, Product4/2
  Product2/1 -> Mux/6
  Product5/1 -> Mux/7
  Demux1/1 -> Gain/1, Product2/1, Product4/1
  Selector/1 -> Trigonometric Function1/1, Trigonometric Function3/1, Trigonometric Function2/1
  ftp/1 -> Selector/1
  Trigonometric Function1/1 -> Demux/1
  Trigonometric Function2/1 -> Demux1/1
  Product4/1 -> Mux/4
  Constant/1 -> Mux/3, Mux/2
  Constant3/1 -> Mux/1
  Trigonometric Function3/1 -> Demux2/1
  pqr/1 -> vrmult/2
  Mux/1 -> vrmult/1
  vrmult/1 -> ftpdot/1

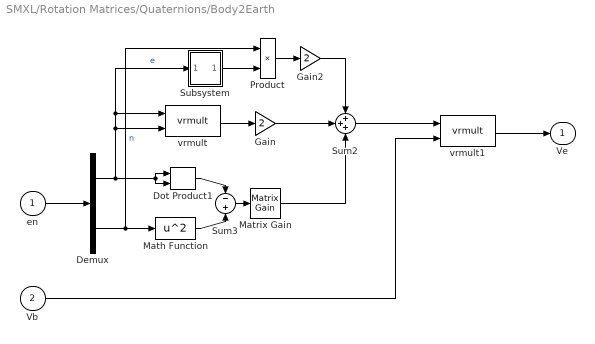
== system SMXL/Rotation Matrices/Quaternions/Body2Earth ==
  en : Inport  Port=1  PortWidth=-1  SampleTime=-1  DataType=auto
      settings: SignalType=auto
  Vb : Inport  Port=2  PortWidth=-1  SampleTime=-1  DataType=auto
      settings: SignalType=auto
  Demux : Demux  Outputs=[3 1]
  Dot Product1 : simulink3/Math/Dot Product
  Gain : Gain  Gain=2  SaturateOnIntegerOverflow=on
  Gain2 : Gain  Gain=2  SaturateOnIntegerOverflow=on
  Math Function : Math  Operator=square  OutputSignalType=auto
  Matrix Gain : simulink3/Math/Matrix Gain  K=[1 0 0 0 1 0 0 0 1]'
  Product : Product  Inputs=2  SaturateOnIntegerOverflow=on
  Subsystem : Subsystem
      mask Display: disp('S')
  Sum2 : Sum  Inputs=+++  SaturateOnIntegerOverflow=on
  Sum3 : Sum  Inputs=-+  SaturateOnIntegerOverflow=on
  vrmult : smxl/Real Matrices/vrmult  dims=[3 1 3]
  vrmult1 : smxl/Real Matrices/vrmult  dims=[3 3 1]
  Ve : Outport  Port=1
  wires:
  vrmult1/1 -> Ve/1
  Vb/1 -> vrmult1/2
  Sum2/1 -> vrmult1/1
  Gain2/1 -> Sum2/1
  Product/1 -> Gain2/1
  Subsystem/1(Out1) -> Product/2
  Demux/2 -> Product/1, Math Function/1  "n"
  Demux/1 -> vrmult/2, vrmult/1, Subsystem/1(In1), Dot Product1/2, Dot Product1/1  "e"
  en/1 -> Demux/1
  Dot Product1/1 -> Sum3/1
  Math Function/1 -> Sum3/2
  Gain/1 -> Sum2/2
  Matrix Gain/1 -> Sum2/3
  vrmult/1 -> Gain/1
  Sum3/1 -> Matrix Gain/1

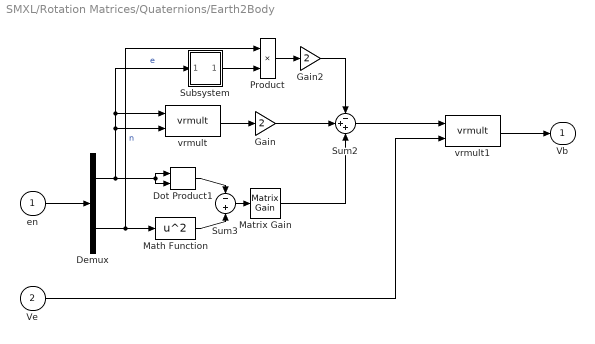
== system SMXL/Rotation Matrices/Quaternions/Earth2Body ==
  en : Inport  Port=1  PortWidth=-1  SampleTime=-1  DataType=auto
      settings: SignalType=auto
  Ve : Inport  Port=2  PortWidth=-1  SampleTime=-1  DataType=auto
      settings: SignalType=auto
  Demux : Demux  Outputs=[3 1]
  Dot Product1 : simulink3/Math/Dot Product
  Gain : Gain  Gain=2  SaturateOnIntegerOverflow=on
  Gain2 : Gain  Gain=2  SaturateOnIntegerOverflow=on
  Math Function : Math  Operator=square  OutputSignalType=auto
  Matrix Gain : simulink3/Math/Matrix Gain  K=[1 0 0 0 1 0 0 0 1]'
  Product : Product  Inputs=2  SaturateOnIntegerOverflow=on
  Subsystem : Subsystem
      mask Display: disp('S')
  Sum2 : Sum  Inputs=-++  SaturateOnIntegerOverflow=on
  Sum3 : Sum  Inputs=-+  SaturateOnIntegerOverflow=on
  vrmult : smxl/Real Matrices/vrmult  dims=[3 1 3]
  vrmult1 : smxl/Real Matrices/vrmult  dims=[3 3 1]
  Vb : Outport  Port=1
  wires:
  Sum3/1 -> Matrix Gain/1
  vrmult/1 -> Gain/1
  Matrix Gain/1 -> Sum2/3
  Gain/1 -> Sum2/2
  Math Function/1 -> Sum3/2
  Dot Product1/1 -> Sum3/1
  en/1 -> Demux/1
  Demux/1 -> Dot Product1/1, Dot Product1/2, Subsystem/1(In1), vrmult/1, vrmult/2  "e"
  Demux/2 -> Math Function/1, Product/1  "n"
  Subsystem/1(Out1) -> Product/2
  Product/1 -> Gain2/1
  Gain2/1 -> Sum2/1
  Sum2/1 -> vrmult1/1
  Ve/1 -> vrmult1/2
  vrmult1/1 -> Vb/1

== system SMXL/Rotation Matrices/Quaternions/endot2pqr ==
  en : Inport  Port=1  PortWidth=-1  SampleTime=-1  DataType=auto
      settings: SignalType=auto
  endot : Inport  Port=2  PortWidth=-1  SampleTime=-1  DataType=auto
      settings: SignalType=auto
  Demux3 : Demux  Outputs=[3 1]
  Gain1 : Gain  Gain=2  SaturateOnIntegerOverflow=on
  Gain2 : Gain  Gain=-1  SaturateOnIntegerOverflow=on
  Mux1 : Mux  Inputs=[9 3]
  Subsystem : Subsystem
      mask Display: disp('S')
  Subsystem1 : Subsystem
      mask Display: disp('I')
  Sum3 : Sum  Inputs=-+  SaturateOnIntegerOverflow=on
  vrmult : smxl/Real Matrices/vrmult  dims=[3 4 1]
  pqr : Outport  Port=1
  wires:
  Demux3/2 -> Subsystem1/1(In1)  "n"
  Subsystem/1(Out1) -> Sum3/1
  Subsystem1/1(Out1) -> Sum3/2
  Demux3/1 -> Subsystem/1(In1), Gain2/1  "e"
  Sum3/1 -> Mux1/1
  Gain1/1 -> vrmult/1
  en/1 -> Demux3/1
  Gain2/1 -> Mux1/2
  Mux1/1 -> Gain1/1
  vrmult/1 -> pqr/1
  endot/1 -> vrmult/2

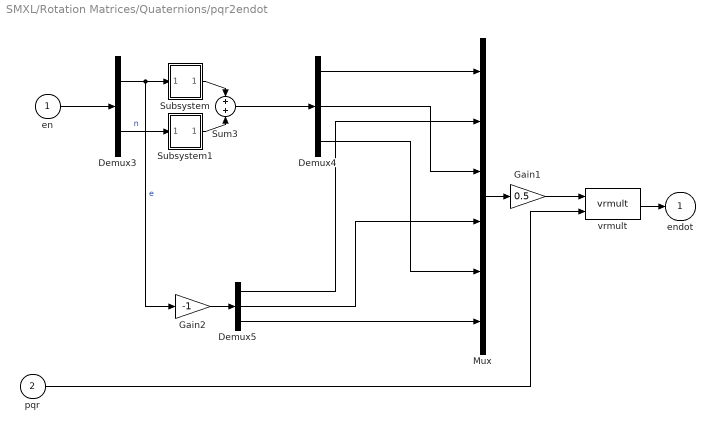
== system SMXL/Rotation Matrices/Quaternions/pqr2endot ==
  en : Inport  Port=1  PortWidth=-1  SampleTime=-1  DataType=auto
      settings: SignalType=auto
  pqr : Inport  Port=2  PortWidth=-1  SampleTime=-1  DataType=auto
      settings: SignalType=auto
  Demux3 : Demux  Outputs=[3 1]
  Demux4 : Demux  Outputs=[3 3 3]
  Demux5 : Demux  Outputs=[1 1 1]
  Gain1 : Gain  Gain=0.5  SaturateOnIntegerOverflow=on
  Gain2 : Gain  Gain=-1  SaturateOnIntegerOverflow=on
  Mux : Mux  Inputs=[3 1 3 1 3 1]
  Subsystem : Subsystem
      mask Display: disp('S')
  Subsystem1 : Subsystem
      mask Display: disp('I')
  Sum3 : Sum  Inputs=++  SaturateOnIntegerOverflow=on
  vrmult : smxl/Real Matrices/vrmult  dims=[4 3 1]
  endot : Outport  Port=1
  wires:
  vrmult/1 -> endot/1
  pqr/1 -> vrmult/2
  en/1 -> Demux3/1
  Demux3/2 -> Subsystem1/1(In1)  "n"
  Subsystem/1(Out1) -> Sum3/1
  Subsystem1/1(Out1) -> Sum3/2
  Demux4/1 -> Mux/1
  Demux3/1 -> Subsystem/1(In1), Gain2/1  "e"
  Gain2/1 -> Demux5/1
  Demux4/2 -> Mux/3
  Demux5/3 -> Mux/6
  Demux5/2 -> Mux/4
  Demux5/1 -> Mux/2
  Demux4/3 -> Mux/5
  Sum3/1 -> Demux4/1
  Mux/1 -> Gain1/1
  Gain1/1 -> vrmult/1

== system SMXL/Rotation Matrices/Euler/Body2Earth/Tcf ==
  theta : Inport  Port=1  PortWidth=-1  SampleTime=-1  DataType=auto
      settings: SignalType=auto
  Constant : Constant  Value=0
  Constant2 : Constant  Value=1
  Gain : Gain  Gain=-1  SaturateOnIntegerOverflow=on
  Mux : Mux  Inputs=9
  Trigonometric Function1 : Trigonometry  Operator=cos  OutputSignalType=auto
  Trigonometric Function2 : Trigonometry  Operator=sin  OutputSignalType=auto
  Tcf : Outport  Port=1
  wires:
  Trigonometric Function1/1 -> Mux/9, Mux/1
  Trigonometric Function2/1 -> Mux/7, Gain/1
  Constant2/1 -> Mux/5
  Constant/1 -> Mux/8, Mux/6, Mux/4, Mux/2
  Gain/1 -> Mux/3
  theta/1 -> Trigonometric Function1/1, Trigonometric Function2/1
  Mux/1 -> Tcf/1

== system SMXL/Rotation Matrices/Euler/Body2Earth/Tfb ==
  phi : Inport  Port=1  PortWidth=-1  SampleTime=-1  DataType=auto
      settings: SignalType=auto
  Constant : Constant  Value=0
  Constant3 : Constant  Value=1
  Gain : Gain  Gain=-1  SaturateOnIntegerOverflow=on
  Mux : Mux  Inputs=9
  Trigonometric Function1 : Trigonometry  Operator=cos  OutputSignalType=auto
  Trigonometric Function2 : Trigonometry  Operator=sin  OutputSignalType=auto
  Tfb : Outport  Port=1
  wires:
  Trigonometric Function1/1 -> Mux/9, Mux/5
  Gain/1 -> Mux/8
  Trigonometric Function2/1 -> Gain/1, Mux/6
  phi/1 -> Trigonometric Function2/1, Trigonometric Function1/1
  Constant/1 -> Mux/7, Mux/4, Mux/3, Mux/2
  Constant3/1 -> Mux/1
  Mux/1 -> Tfb/1

== system SMXL/Rotation Matrices/Euler/Body2Earth/Toc ==
  psi : Inport  Port=1  PortWidth=-1  SampleTime=-1  DataType=auto
      settings: SignalType=auto
  Constant : Constant  Value=0
  Constant2 : Constant  Value=1
  Gain : Gain  Gain=-1  SaturateOnIntegerOverflow=on
  Mux : Mux  Inputs=9
  Trigonometric Function1 : Trigonometry  Operator=cos  OutputSignalType=auto
  Trigonometric Function2 : Trigonometry  Operator=sin  OutputSignalType=auto
  Toc : Outport  Port=1
  wires:
  Mux/1 -> Toc/1
  Constant/1 -> Mux/6, Mux/8, Mux/7, Mux/3
  Constant2/1 -> Mux/9
  Gain/1 -> Mux/4
  Trigonometric Function2/1 -> Mux/2, Gain/1
  Trigonometric Function1/1 -> Mux/5, Mux/1
  psi/1 -> Trigonometric Function2/1, Trigonometric Function1/1

== system SMXL/Rotation Matrices/Euler/Body2Wind/Tcf ==
  alpha : Inport  Port=1  PortWidth=-1  SampleTime=-1  DataType=auto
      settings: SignalType=auto
  Constant : Constant  Value=0
  Constant2 : Constant  Value=1
  Gain : Gain  Gain=-1  SaturateOnIntegerOverflow=on
  Mux : Mux  Inputs=9
  Trigonometric Function1 : Trigonometry  Operator=cos  OutputSignalType=auto
  Trigonometric Function2 : Trigonometry  Operator=sin  OutputSignalType=auto
  Tcf : Outport  Port=1
  wires:
  Trigonometric Function1/1 -> Mux/9, Mux/1
  Trigonometric Function2/1 -> Mux/7, Gain/1
  Constant2/1 -> Mux/5
  Constant/1 -> Mux/8, Mux/6, Mux/4, Mux/2
  Gain/1 -> Mux/3
  alpha/1 -> Trigonometric Function1/1, Trigonometric Function2/1
  Mux/1 -> Tcf/1

== system SMXL/Rotation Matrices/Euler/Body2Wind/Toc ==
  beta : Inport  Port=1  PortWidth=-1  SampleTime=-1  DataType=auto
      settings: SignalType=auto
  Constant : Constant  Value=0
  Constant2 : Constant  Value=1
  Gain : Gain  Gain=-1  SaturateOnIntegerOverflow=on
  Mux : Mux  Inputs=9
  Trigonometric Function1 : Trigonometry  Operator=cos  OutputSignalType=auto
  Trigonometric Function2 : Trigonometry  Operator=sin  OutputSignalType=auto
  Toc : Outport  Port=1
  wires:
  Mux/1 -> Toc/1
  Constant/1 -> Mux/6, Mux/8, Mux/7, Mux/3
  Constant2/1 -> Mux/9
  Gain/1 -> Mux/4
  Trigonometric Function2/1 -> Mux/2, Gain/1
  Trigonometric Function1/1 -> Mux/5, Mux/1
  beta/1 -> Trigonometric Function2/1, Trigonometric Function1/1

== system SMXL/Rotation Matrices/Euler/Earth2Body/Tcf ==
  theta : Inport  Port=1  PortWidth=-1  SampleTime=-1  DataType=auto
      settings: SignalType=auto
  Constant : Constant  Value=0
  Constant2 : Constant  Value=1
  Gain : Gain  Gain=-1  SaturateOnIntegerOverflow=on
  Mux : Mux  Inputs=9
  Trigonometric Function1 : Trigonometry  Operator=cos  OutputSignalType=auto
  Trigonometric Function2 : Trigonometry  Operator=sin  OutputSignalType=auto
  Tcf : Outport  Port=1
  wires:
  Mux/1 -> Tcf/1
  theta/1 -> Trigonometric Function2/1, Trigonometric Function1/1
  Gain/1 -> Mux/3
  Constant/1 -> Mux/2, Mux/4, Mux/6, Mux/8
  Constant2/1 -> Mux/5
  Trigonometric Function2/1 -> Gain/1, Mux/7
  Trigonometric Function1/1 -> Mux/1, Mux/9

== system SMXL/Rotation Matrices/Euler/Earth2Body/Tfb ==
  phi : Inport  Port=1  PortWidth=-1  SampleTime=-1  DataType=auto
      settings: SignalType=auto
  Constant : Constant  Value=0
  Constant3 : Constant  Value=1
  Gain : Gain  Gain=-1  SaturateOnIntegerOverflow=on
  Mux : Mux  Inputs=9
  Trigonometric Function1 : Trigonometry  Operator=cos  OutputSignalType=auto
  Trigonometric Function2 : Trigonometry  Operator=sin  OutputSignalType=auto
  Tfb : Outport  Port=1
  wires:
  Mux/1 -> Tfb/1
  Constant3/1 -> Mux/1
  Constant/1 -> Mux/2, Mux/3, Mux/4, Mux/7
  phi/1 -> Trigonometric Function1/1, Trigonometric Function2/1
  Trigonometric Function2/1 -> Mux/6, Gain/1
  Gain/1 -> Mux/8
  Trigonometric Function1/1 -> Mux/5, Mux/9

== system SMXL/Rotation Matrices/Euler/Earth2Body/Toc ==
  psi : Inport  Port=1  PortWidth=-1  SampleTime=-1  DataType=auto
      settings: SignalType=auto
  Constant : Constant  Value=0
  Constant2 : Constant  Value=1
  Gain : Gain  Gain=-1  SaturateOnIntegerOverflow=on
  Mux : Mux  Inputs=9
  Trigonometric Function1 : Trigonometry  Operator=cos  OutputSignalType=auto
  Trigonometric Function2 : Trigonometry  Operator=sin  OutputSignalType=auto
  Toc : Outport  Port=1
  wires:
  psi/1 -> Trigonometric Function1/1, Trigonometric Function2/1
  Trigonometric Function1/1 -> Mux/1, Mux/5
  Trigonometric Function2/1 -> Gain/1, Mux/2
  Gain/1 -> Mux/4
  Constant2/1 -> Mux/9
  Constant/1 -> Mux/3, Mux/7, Mux/8, Mux/6
  Mux/1 -> Toc/1

== system SMXL/Rotation Matrices/Euler/Earth2Kine/Tcf ==
  gamma : Inport  Port=1  PortWidth=-1  SampleTime=-1  DataType=auto
      settings: SignalType=auto
  Constant : Constant  Value=0
  Constant2 : Constant  Value=1
  Gain : Gain  Gain=-1  SaturateOnIntegerOverflow=on
  Mux : Mux  Inputs=9
  Trigonometric Function1 : Trigonometry  Operator=cos  OutputSignalType=auto
  Trigonometric Function2 : Trigonometry  Operator=sin  OutputSignalType=auto
  Tcf : Outport  Port=1
  wires:
  Trigonometric Function1/1 -> Mux/9, Mux/1
  Trigonometric Function2/1 -> Mux/7, Gain/1
  Constant2/1 -> Mux/5
  Constant/1 -> Mux/8, Mux/6, Mux/4, Mux/2
  Gain/1 -> Mux/3
  gamma/1 -> Trigonometric Function1/1, Trigonometric Function2/1
  Mux/1 -> Tcf/1
